simulink model "BalanceMIPS"  (R2022b)
settings: Solver=FixedStepDiscrete  StartTime=0.0  StopTime=.8  RelTol=1e-3  EnableMultiTasking=on
InitFcn:
  | % Initialize model
  | run('BalanceMIPSInit.m');
  | 
  | % load library data
  | GainLibrary_data;
model workspace (MAT data in the model file):
  PreampVolumeTable_Idx = Simulink.Signal
  PreampVolumeTable_Idx.DataType = 'auto'
  PreampVolumeTable_Idx.Dimensions = -1
  PreampVolumeTable_Idx.DimensionsMode = 'auto'
  PreampVolumeTable_Idx.Complexity = 'auto'
  PreampVolumeTable_Idx.SampleTime = -1
  PreampVolumeTable_Idx.SamplingMode = 'auto'
  PreampVolumeTable_Idx.InitialValue = 'uint8([0 255 255 255 255 255])'
  Range = Simulink.Signal
  Range.DataType = 'auto'
  Range.Dimensions = -1
  Range.DimensionsMode = 'auto'
  Range.Complexity = 'auto'
  Range.SampleTime = -1
  Range.SamplingMode = 'auto'
  Table_Idx = Simulink.Signal
  Table_Idx.DataType = 'auto'
  Table_Idx.Dimensions = -1
  Table_Idx.DimensionsMode = 'auto'
  Table_Idx.Complexity = 'auto'
  Table_Idx.SampleTime = -1
  Table_Idx.SamplingMode = 'auto'
values from neighbouring files (symbols this model uses):
  frame_size = 32    [BalanceMIPSInit.m]
undefined symbols (not defined in the file or in its folder): carModel, mode, numChannel, sampleRate
libraries: FeaturePath x1, Balance x1
settings Model: Creator=sk1042978  LastModifiedBy=kl13806
settings SolverCC: AlgebraicLoopSolver=TrustRegion
settings OptimizationCC: DefaultParameterBehavior=Inlined  DefaultUnderspecifiedDataType=single  EfficientTunableParamExpr=on
settings DebuggingCC: InheritedTsInSrcMsg=none  MultiTaskDSMMsg=none  ParameterPrecisionLossMsg=none  ParameterTunabilityLossMsg=error  UnconnectedInputMsg=warning  UnconnectedOutputMsg=warning  UnconnectedLineMsg=warning  UnknownTsInhSupMsg=none  SFUnexpectedBacktrackingDiag=warning  SFNoUnconditionalDefaultTransitionDiag=warning  SFExecutionAtInitializationDiag=none  SFMachineParentedDataDiag=warning  ArithmeticOperatorsInVariantConditions=warning
settings HardwareCC: ProdBitPerPointer=32  ProdBitPerSizeT=32  ProdBitPerPtrDiffT=32  ProdWordSize=32  ProdHWDeviceType=Intel->x86-32 (Windows32)  TargetBitPerPointer=64  TargetBitPerSizeT=64  TargetBitPerPtrDiffT=64  TargetLongLongMode=on  TargetIntDivRoundTo=Zero  TargetEndianess=LittleEndian  TargetWordSize=64  TargetHWDeviceType=MATLAB Host  ProdEqTarget=off
settings ModelReferenceCC: EnableRefExpFcnMdlSchedulingChecks=on
settings SFSimCC: SimUseLocalCustomCode=off  MATLABDynamicMemAlloc=off  CustomCodeUndefinedFunction=UseInterfaceOnly
settings RTWCC: Description=Embedded Coder (host-based shared library target)  SystemTargetFile=ert_shrlib.tlc  GenCodeOnly=on  TemplateMakefile=ert_default_tmf  GenerateReport=on  RetainRTWFile=on  RTWUseLocalCustomCode=off  Toolchain=MinGW64 | gmake (64-bit Windows)  BuildConfiguration=Faster Runs  IncludeHyperlinkInReport=on  LaunchReport=on  GenerateTraceInfo=on  GenerateTraceReport=on  GenerateTraceReportSl=on  GenerateTraceReportSf=on  GenerateTraceReportEml=on  GenerateCodeMetricsReport=on  DLArmComputeVersion=19.05
settings CodeAppCC: ForceParamTrailComments=on  IgnoreCustomStorageClasses=off  OperatorAnnotations=on  SimulinkDataObjDesc=on  SFDataObjDesc=on  MATLABFcnDesc=on  InsertBlockDesc=on  StateflowObjectComments=on  MATLABSourceComments=on
settings STFCustomTargetCC: TargetLangStandard=C99 (ISO)  ParMdlRefBuildCompliant=on  CompOptLevelCompliant=on  CombineOutputUpdateFcns=on  ERTCustomFileBanners=on  SupportContinuousTime=off  SupportNonInlinedSFcns=off  RemoveResetFunc=on  SupportVariableSizeSignals=on  MATLABClassNameForMDSCustomization=Simulink.SoftwareTarget.ERTCustomization  ModelStepFunctionPrototypeControlCompliant=on  UseToolchainInfoCompliant=on  SystemTargetFile=ert_shrlib.tlc
settings ERTTargetCC: TargetLangStandard=C99 (ISO)  MultiwordLength=2048  ConcurrentExecutionCompliant=off  SupportVariableSizeSignals=on  CPPClassGenCompliant=off  InlinedParameterPlacement=NonHierarchical  ERTCustomFileTemplate=example_file_process.tlc
settings ConfigComp: CovMetricSettings=dw  CovSaveCumulativeToWorkspaceVar=on  CovSaveSingleToWorkspaceVar=on  CovExternalEMLEnable=off

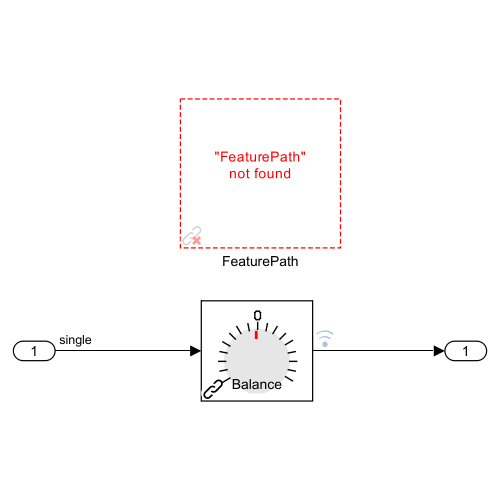
[thumbnail: Simulink's stored preview of the top-level diagram]
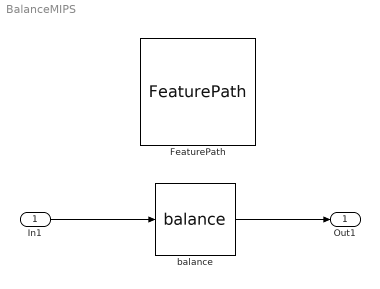
== system BalanceMIPS ==
  In1 : Inport  OutDataTypeStr=single  PortDimensions=[frame_size numChannel]  SampleTime=1/sampleRate*frame_size
  FeaturePath : FeaturePath/FeaturePath  FeatureName=BalanceMIPS  IsGroup=on  GroupNumber=-1  DeclarePackages=off  PackageNames=mode,carModel  IsModule=off  TriggerInit=[80 -386 195 -279]
  balance : Balance/balance  BankNumber=0  MaskFeatureName=Balance  MaskOffset=128  MaskChanRampMap=channelMap  MaskSilentExtreme=on  MaskSilentExtremeBass=off  MaskBoostDisable=off
  Out1 : Outport  VectorParamsAs1DForOutWhenUnconnected=off
  wires:
  balance/1 -> Out1/1
  In1/1 -> balance/1
